simulink model "twolinkarm_pd"  (R2017a)
settings: Solver=FixedStepAuto  StartTime=0.0  StopTime=10.0  FixedStep=0.001  MaxStep=0.01  RelTol=1e-4  AbsTol=1e-3
InitFcn:
  | twolinkarm_init
values from neighbouring files (symbols this model uses):
  delayTime1 = 0    [twolinkarm_init.m]
  delayTime2 = 0    [twolinkarm_init.m]
  g = 9.81    [twolinkarm_init.m]
  J2 = m2*l2^2/3    (= 0.213333333333)    [twolinkarm_init.m]
  Kd1 = 50    [twolinkarm_init.m]
  Kd2 = 50    [twolinkarm_init.m]
  Kp1 = 100    [twolinkarm_init.m]
  Kp2 = 100    [twolinkarm_init.m]
  l1 = 2*l1    [twolinkarm_draw_save_animation.m]    (also in twolinkarm_init.m = 1)
  l2 = 2*l2    [twolinkarm_draw_save_animation.m]    (also in twolinkarm_init.m = 0.8)
  m1 = 1    [twolinkarm_init.m]
  m2 = 1    [twolinkarm_init.m]
  q_desired = [0;0;0;0]    [run_twolinkarm_lqr.m]    (also in run_twolinkarm_nonlinear_numerical.m = [pi/2;2*pi/3;0;0]; run_twolinkarm_simulink.m = [pi/4;pi/5;0;0])
  q_init = [-pi/2;0;0;0]    [run_twolinkarm_lqr.m]    (also in run_twolinkarm_nonlinear_numerical.m = [-pi/4;-pi/4;0;0]; run_twolinkarm_simulink.m)
settings Model: Creator=Lingfeng Sun  LastModifiedBy=Lingfeng Sun
settings SolverCC: MaxConsecutiveMinStep=10

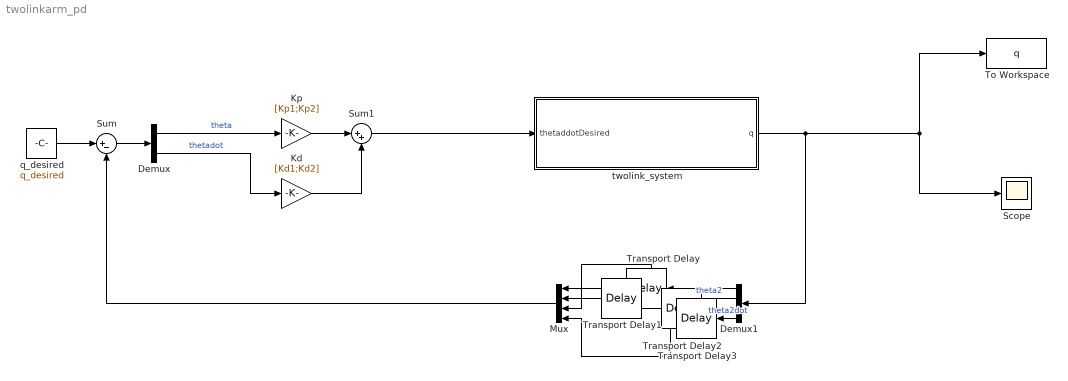
== system twolinkarm_pd ==
  Demux : Demux  Outputs=2
  Demux1 : Demux
  Kd : Gain  Gain=[Kd1;Kd2]
  Kp : Gain  Gain=[Kp1;Kp2]
  Mux : Mux
  Scope : Scope
  Sum : Sum  Inputs=|+-
  Sum1 : Sum  Inputs=|++
  To Workspace : ToWorkspace  VariableName=q  SaveFormat=Timeseries  SampleTime=-1
  Transport Delay : TransportDelay  DelayTime=delayTime1
  Transport Delay1 : TransportDelay  DelayTime=delayTime2
  Transport Delay2 : TransportDelay  DelayTime=delayTime1
  Transport Delay3 : TransportDelay  DelayTime=delayTime2
  q_desired : Constant  Value=q_desired
  twolink_system : Subsystem
  wires:
  q_desired/1 -> Sum/1
  twolink_system/1(q) -> Demux1/1, Scope/1, To Workspace/1
  Sum/1 -> Demux/1
  Demux/1 -> Kp/1  "theta"
  Demux/2 -> Kd/1  "thetadot"
  Kp/1 -> Sum1/1
  Kd/1 -> Sum1/2
  Sum1/1 -> twolink_system/1("thetaddotDesired ")
  Mux/1 -> Sum/2
  Demux1/2 -> Transport Delay1/1  "theta2"
  Demux1/4 -> Transport Delay3/1  "theta2dot"
  Demux1/1 -> Transport Delay/1
  Demux1/3 -> Transport Delay2/1
  Transport Delay/1 -> Mux/1
  Transport Delay2/1 -> Mux/3
  Transport Delay1/1 -> Mux/2
  Transport Delay3/1 -> Mux/4

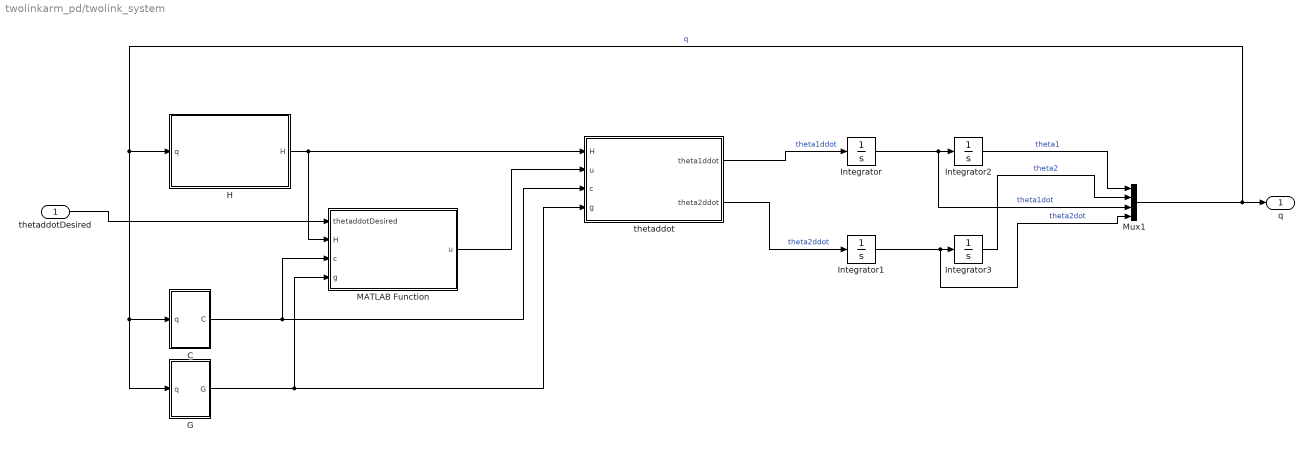
== system twolinkarm_pd/twolink_system ==
  "thetaddotDesired " : Inport  PortDimensions=[2 1]
  C : Subsystem
  G : Subsystem
  H : Subsystem
  Integrator : Integrator  InitialCondition=q_init(3)
  Integrator1 : Integrator  InitialCondition=q_init(4)
  Integrator2 : Integrator  InitialCondition=q_init(1)
  Integrator3 : Integrator  InitialCondition=q_init(2)
  MATLAB Function : MATLAB Function  TreatAsAtomicUnit=on
  Mux1 : Mux
  thetaddot : MATLAB Function  TreatAsAtomicUnit=on
  q : Outport
  wires:
  Integrator1/1 -> Mux1/4, Integrator3/1  "theta2dot"
  Integrator/1 -> Mux1/3, Integrator2/1  "theta1dot"
  H/1(H) -> MATLAB Function/2(H), thetaddot/1(H)
  "thetaddotDesired "/1 -> MATLAB Function/1(thetaddotDesired)
  C/1(C) -> MATLAB Function/3(c), thetaddot/3(c)
  G/1(G) -> MATLAB Function/4(g), thetaddot/4(g)
  thetaddot/1(theta1ddot) -> Integrator/1  "theta1ddot"
  thetaddot/2(theta2ddot) -> Integrator1/1  "theta2ddot"
  Mux1/1 -> C/1(q), G/1(q), H/1(q), q/1  "q"
  Integrator2/1 -> Mux1/1  "theta1"
  Integrator3/1 -> Mux1/2  "theta2"
  MATLAB Function/1(u) -> thetaddot/2(u)

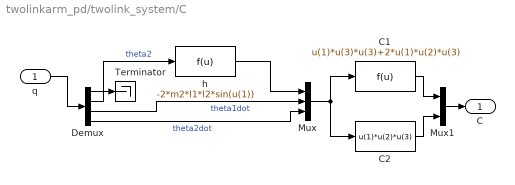
== system twolinkarm_pd/twolink_system/C ==
  q : Inport  PortDimensions=[4 1]
  C1 : Fcn  Expr=u(1)*u(3)*u(3)+2*u(1)*u(2)*u(3)
  C2 : Fcn  Expr=u(1)*u(2)*u(3)
  Demux : Demux
  Mux : Mux  Inputs=3
  Mux1 : Mux  Inputs=2
  Terminator : Terminator
  h : Fcn  Expr=-2*m2*l1*l2*sin(u(1))
  C : Outport
  wires:
  q/1 -> Demux/1
  Mux/1 -> C2/1, C1/1
  Demux/3 -> Mux/2  "theta1dot"
  Demux/4 -> Mux/3  "theta2dot"
  Demux/2 -> h/1  "theta2"
  h/1 -> Mux/1
  Mux1/1 -> C/1
  C1/1 -> Mux1/1
  C2/1 -> Mux1/2
  Demux/1 -> Terminator/1

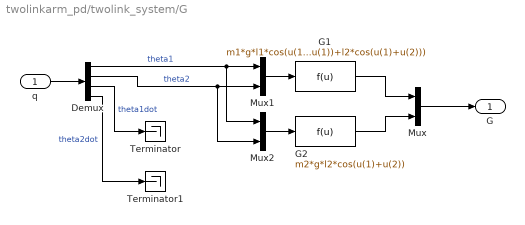
== system twolinkarm_pd/twolink_system/G ==
  q : Inport  PortDimensions=[4 1]
  Demux : Demux
  G1 : Fcn  Expr=m1*g*l1*cos(u(1))+m2*g*(2*l1*cos(u(1))+l2*cos(u(1)+u(2)))
  G2 : Fcn  Expr=m2*g*l2*cos(u(1)+u(2))
  Mux : Mux  Inputs=2
  Mux1 : Mux  Inputs=2
  Mux2 : Mux  Inputs=2
  Terminator : Terminator
  Terminator1 : Terminator
  G : Outport
  wires:
  G1/1 -> Mux/1
  G2/1 -> Mux/2
  q/1 -> Demux/1
  Mux1/1 -> G1/1
  Mux2/1 -> G2/1
  Demux/1 -> Mux2/1, Mux1/1  "theta1"
  Demux/2 -> Mux2/2, Mux1/2  "theta2"
  Mux/1 -> G/1
  Demux/3 -> Terminator/1  "theta1dot"
  Demux/4 -> Terminator1/1  "theta2dot"

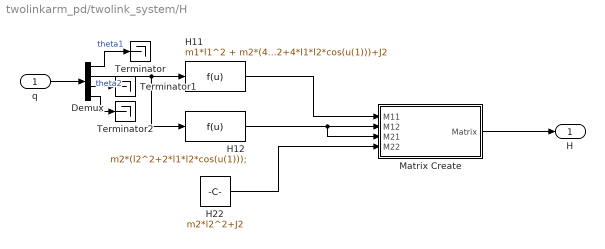
== system twolinkarm_pd/twolink_system/H ==
  q : Inport  PortDimensions=[4 1]
  Demux : Demux
  H11 : Fcn  Expr=m1*l1^2 + m2*(4*l1^2+l2^2+4*l1*l2*cos(u(1)))+J2
  H12 : Fcn  Expr=m2*(l2^2+2*l1*l2*cos(u(1)));
  H22 : Constant  Value=m2*l2^2+J2
  Matrix Create : Subsystem
  Terminator : Terminator
  Terminator1 : Terminator
  Terminator2 : Terminator
  H : Outport  PortDimensions=[2 2]
  wires:
  H11/1 -> Matrix Create/1(M11)
  H22/1 -> Matrix Create/4(M22)
  H12/1 -> Matrix Create/3(M21), Matrix Create/2(M12)
  Matrix Create/1(Matrix) -> H/1
  q/1 -> Demux/1
  Demux/2 -> H12/1, H11/1  "theta2"
  Demux/1 -> Terminator/1  "theta1"
  Demux/3 -> Terminator1/1
  Demux/4 -> Terminator2/1

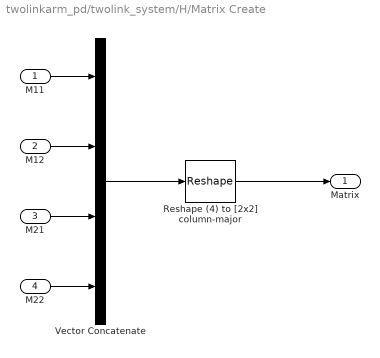
== system twolinkarm_pd/twolink_system/H/Matrix Create ==
  M11 : Inport  PortDimensions=1
  M12 : Inport  Port=2  PortDimensions=1
  M21 : Inport  Port=3  PortDimensions=1
  M22 : Inport  Port=4  PortDimensions=1
  Reshape (4) to [2x2] column-major : Reshape  OutputDimensionality=Customize  OutputDimensions=[2,2]
  Vector Concatenate : Concatenate  NumInputs=4
  Matrix : Outport
  wires:
  Reshape (4) to [2x2] column-major/1 -> Matrix/1
  M11/1 -> Vector Concatenate/1
  Vector Concatenate/1 -> Reshape (4) to [2x2] column-major/1
  M12/1 -> Vector Concatenate/2
  M21/1 -> Vector Concatenate/3
  M22/1 -> Vector Concatenate/4

== matlab function twolinkarm_pd/twolink_system/MATLAB Function ==
  data: thetaddotDesired input; u output; H input; c input; g input
function u = fcn(thetaddotDesired,H,c,g)
u = thetaddotDesired;

== matlab function twolinkarm_pd/twolink_system/thetaddot ==
  data: H input; u input; theta1ddot output; c input; g input; theta2ddot output
function [theta1ddot,theta2ddot] = theta(H,u,c,g)
S = H^(-1)*(u-c-g);
theta1ddot = S(1);
theta2ddot = S(2);
end
